simulink library "RF"  (Simulink 4.00)
values from neighbouring files (symbols this model uses):
  A = rms(interp1(f,MX,fb))    [fftbandamp.m]    (also in logfft.m = fftamp(samples, fs, f, varargin{:})/vpp; plotfft.m = fftamp(samples, fs, f, varargin{:})*2/vpp)
  P = sinc((1575.42 - f)/10.23).^2./10.23    [L1PSD.m]    (also in fftphase.m = interp1(f,PX,f0))
undefined symbols (not defined in the file or in its folder): adb, B, CA_ID, fs, j, m, N, p, Phi, Range, Rice_K, Rice_Seed, Rice_Sigma, tau_delay, z
libraries: RF x133, dspcmplx x47, com_sour x8, dspelmat x8, com_chan x4, dspbdsp x3, dspswit x3, simulink_extras x2, com_filt x2
(part 2 of 5)

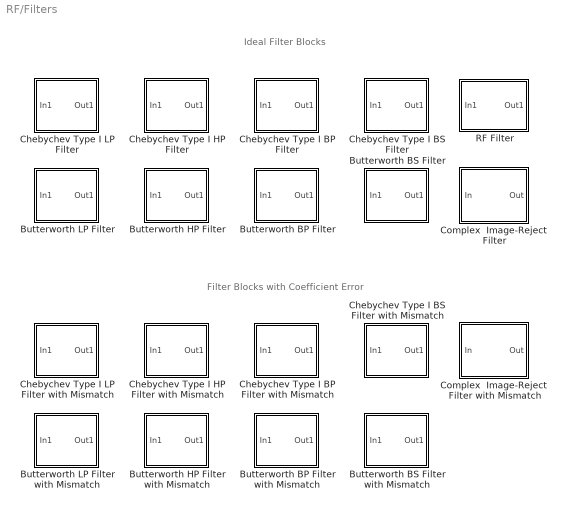
== system RF/Filters ==
  note: Ideal Filter Blocks
  note: Filter Blocks with Coefficient Error
  Butterworth BP Filter : Subsystem  mask(Butterworth Bandpass Filter){w1=200*2*pi, w2=300*2*pi, order=4}
      mask prompts: w1 "Lower Cutoff frequency (rad/sec):"; w2 "Upper Cutoff Frequency"
      mask help: Analog Butterworth bandpass filter.
      mask init:
      | [num,den]=butter(floor(order/2),[w1 w2],'s'); [z,p,k]=tf2zp(num,den); w=logspace(log10(w1/10),log10(10*w2),50);
      | k=k/max(abs(freqs(num,den,w)));[num,den]=zp2tf(z,p,k);h=freqs(num,den,w);
      settings: RTWFcnNameOpts=Auto  RTWFileNameOpts=Auto
      mask Help: Analog Butterworth bandpass filter.
      mask Display: plot(20*log10(w),20*log10(abs(h)))
  Butterworth BP Filter with Mismatch : Subsystem  mask(Butterworth Bandpass Filter with Mismatch){w1=200*2*pi, w2=300*2*pi, order=4, ErrorStd=1}
      mask prompts: w1 "Lower Cutoff frequency (rad/sec):"; w2 "Upper Cutoff Frequency"; ErrorStd "Coefficient Standard Error (Percent Nominal Value)"
      mask help: Analog Butterworth bandpass filter. Coefficient Error is modeled as percent nominal value error.
      mask init:
      | [num,den]=butter(floor(order/2),[w1 w2],'s');[z,p,k]=tf2zp(num,den);
      | w=logspace(log10(w1/10),log10(10*w2),50);
      | k=k/max(abs(freqs(num,den,w))); [num,den]=zp2tf(z,p,k);
      | num = num + num .* ErrorStd/100 .* randn(1,length(num));
      | den = den + den .* ErrorStd/100 .* randn(1,length(den));
      | [z,p,k]=tf2zp(num,den); h=freqs(num,den,w);
      settings: RTWFcnNameOpts=Auto  RTWFileNameOpts=Auto
      mask Help: Analog Butterworth bandpass filter.  Coefficient Error is modeled as percent nominal value error.
      mask Display: plot(20*log10(w),20*log10(abs(h)))
  Butterworth BS Filter : Subsystem  mask(Butterworth Bandstop Filter){w1=100*2*pi, w2=200*2*pi, order=4}
      mask prompts: w1 "Lower Cutoff frequency (rad/sec):"; w2 "Upper Cutoff frequency (rad/sec)"
      mask help: Analog Butterworth bandstop filter.
      mask init:
      | [num,den]=butter(floor(order/2),[w1 w2],'stop','s');[z,p,k]=tf2zp(num,den);
      | w=logspace(log10(w1/10),log10(10*w2),50);
      | k=k/max(abs(freqs(num,den,w)));[num,den]=zp2tf(z,p,k);h=freqs(num,den,w);
      settings: RTWFcnNameOpts=Auto  RTWFileNameOpts=Auto
      mask Help: Analog Butterworth bandstop filter.
      mask Display: plot(20*log10(w),20*log10(abs(h)))
  Butterworth BS Filter with Mismatch : Subsystem  mask(Butterworth Bandstop Filter with Mismatch){w1=100*2*pi, w2=200*2*pi, order=4, ErrorStd=1}
      mask prompts: w1 "Lower Cutoff frequency (rad/sec):"; w2 "Upper Cutoff frequency (rad/sec)"; ErrorStd "Coefficient Standard Error (Percent Nominal Value)"
      mask help: Analog Butterworth bandstop filter. Coefficient Error is modeled as percent nominal value error.
      mask init:
      | [num,den]=butter(floor(order/2),[w1 w2],'stop','s');[z,p,k]=tf2zp(num,den);
      | w=logspace(log10(w1/10),log10(10*w2),50);
      | k=k/max(abs(freqs(num,den,w)));[num,den]=zp2tf(z,p,k);
      | num = num + num .* ErrorStd/100 .* randn(1,length(num));
      | den = den + den .* ErrorStd/100 .* randn(1,length(den));
      | [z,p,k]=tf2zp(num,den); h=freqs(num,den,w);
      settings: RTWFcnNameOpts=Auto  RTWFileNameOpts=Auto
      mask Help: Analog Butterworth bandstop filter.  Coefficient Error is modeled as percent nominal value error.
      mask Display: plot(20*log10(w),20*log10(abs(h)))
  Butterworth HP Filter : Subsystem  mask(Butterworth Highpass Filter){w0=100*2*pi, order=4}
      mask prompts: w0 "Cutoff frequency (rad/sec):"
      mask help: Analog Butterworth highpass filter.
      mask init:
      | [num,den]=butter(order,w0,'high','s');[z,p,k]=tf2zp(num,den);
      | w=logspace(log10(w0/10),log10(10*w0),50);
      | k=k/max(abs(freqs(num,den,w)));[num,den]=zp2tf(z,p,k);h=freqs(num,den,w);
      settings: RTWFcnNameOpts=Auto  RTWFileNameOpts=Auto
      mask Help: Analog Butterworth highpass filter.
      mask Display: plot(20*log10(w),20*log10(abs(h)))
  Butterworth HP Filter with Mismatch : Subsystem  mask(Butterworth Highpass Filter with Mismatch){w0=100*2*pi, order=4, ErrorStd=1}
      mask prompts: w0 "Cutoff frequency (rad/sec):"; ErrorStd "Coefficient Standard Error (Percent Nominal Value)"
      mask help: Analog Butterworth highpass filter. Coefficient Error is modeled as percent nominal value error.
      mask init:
      | [num,den]=butter(order,w0,'high','s');[z,p,k]=tf2zp(num,den);
      | w=logspace(log10(w0/10),log10(10*w0),50);
      | k=k/max(abs(freqs(num,den,w))); [num,den]=zp2tf(z,p,k);
      | num = num + num .* ErrorStd/100 .* randn(1,length(num));
      | den = den + den .* ErrorStd/100 .* randn(1,length(den));
      | [z,p,k]=tf2zp(num,den); h=freqs(num,den,w);
      settings: RTWFcnNameOpts=Auto  RTWFileNameOpts=Auto
      mask Help: Analog Butterworth highpass filter.  Coefficient Error is modeled as percent nominal value error.
      mask Display: plot(20*log10(w),20*log10(abs(h)))
  Butterworth LP Filter : Subsystem  mask(Butterworth Lowpass Filter){w0=100*2*pi, order=4}
      mask prompts: w0 "Cutoff frequency (rad/sec):"
      mask help: Analog Butterworth low pass filter.
      mask init:
      | [num,den]=butter(order,w0,'s');[z,p,k]=tf2zp(num,den);
      | w=logspace(log10(w0/10),log10(10*w0),50);
      | k=k/max(abs(freqs(num,den,w)));[num,den]=zp2tf(z,p,k); h=freqs(num,den,w);
      settings: RTWFcnNameOpts=Auto  RTWFileNameOpts=Auto
      mask Help: Analog Butterworth low pass filter.
      mask Display: plot(20*log10(w),20*log10(abs(h)))
  Butterworth LP Filter with Mismatch : Subsystem  mask(Butterworth Lowpass Filter with Mismatch){w0=100*2*pi, order=4, ErrorStd=1}
      mask prompts: w0 "Cutoff frequency (rad/sec):"; ErrorStd "Coefficient Standard Error (Percent Nominal Value)"
      mask help: Analog Butterworth low pass filter. Coefficient Error is modeled as percent nominal value error.
      mask init:
      | [num,den]=butter(order,w0,'s');[z,p,k]=tf2zp(num,den);
      | w=logspace(log10(w0/10),log10(10*w0),50);
      | k=k/max(abs(freqs(num,den,w)));[num,den]=zp2tf(z,p,k);
      | num = num + num .* ErrorStd/100 .* randn(1,length(num));
      | den = den + den .* ErrorStd/100 .* randn(1,length(den));
      | [z,p,k]=tf2zp(num,den); h=freqs(num,den,w);
      settings: RTWFcnNameOpts=Auto  RTWFileNameOpts=Auto
      mask Help: Analog Butterworth low pass filter.  Coefficient Error is modeled as percent nominal value error.
      mask Display: plot(20*log10(w),20*log10(abs(h)))
  Chebychev Type I BP Filter : Subsystem  mask(Chebychev Type I Bandpass Filter){w1=200*2*pi, w2=300*2*pi, order=4, ripple=0.5}
      mask prompts: w1 "Lower Cutoff frequency (rad/sec):"; w2 "Upper Cutoff frequency (rad/sec)"; ripple "Db ripple in passband:"
      mask help: Analog Chebyshev type I bandpass filter.
      mask init:
      | [z,p,k]=cheby1(floor(order/2),ripple,[w1 w2],'s');
      | [num,den]=zp2tf(z,p,1); w=logspace(log10(w1/10),log10(10*w2),50);
      | k = 1/max(abs(freqs(num,den,w)));[num,den]=zp2tf(z,p,k);
      | h=freqs(num,den,w);
      settings: RTWFcnNameOpts=Auto  RTWFileNameOpts=Auto
      mask Help: Analog Chebyshev type I bandpass filter.
      mask Display: plot(20*log10(w),20*log10(abs(h)))
  Chebychev Type I BP Filter with Mismatch : Subsystem  mask(Chebychev Type I Bandpass Filter with Mismatch){w1=200*2*pi, w2=300*2*pi, order=4, ripple=0.5, ErrorStd=1}
      mask prompts: w1 "Lower Cutoff frequency (rad/sec):"; w2 "Upper Cutoff frequency (rad/sec)"; ripple "Db ripple in passband:"; ErrorStd "Coefficient Standard Error (Percent Nominal Value)"
      mask help: Analog Chebyshev type I bandpass filter. Coefficient Error is modeled as percent nominal value error.
      mask init:
      | [z,p,k]=cheby1(floor(order/2),ripple,[w1 w2],'s');
      | [num,den]=zp2tf(z,p,1); w=logspace(log10(w1/10),log10(10*w2),50);
      | k = 1/max(abs(freqs(num,den,w)));[num,den]=zp2tf(z,p,k);
      | num = num + num .* ErrorStd/100 .* randn(1,length(num));
      | den = den + den .* ErrorStd/100 .* randn(1,length(den));
      | [z,p,k]=tf2zp(num,den); h=freqs(num,den,w);
      settings: RTWFcnNameOpts=Auto  RTWFileNameOpts=Auto
      mask Help: Analog Chebyshev type I bandpass filter.  Coefficient Error is modeled as percent nominal value error.
      mask Display: plot(20*log10(w),20*log10(abs(h)))
  Chebychev Type I BS Filter : Subsystem  mask(Chebychev Type I Bandstop Filter){w1=100*2*pi, w2=200*2*pi, order=4, ripple=0.5}
      mask prompts: w1 "Lower Cutoff frequency (rad/sec):"; w2 "Upper Cutoff frequency (rad/sec)"; ripple "Db ripple in passband:"
      mask help: Analog Chebyshev type I bandstop filter.
      mask init:
      | [z,p,k]=cheby1(floor(order/2),ripple,[w1 w2],'stop','s');
      |  w=logspace(log10(w1/10),log10(10*w2),50);[num,den]=zp2tf(z,p,1);
      | k =1/max(abs(freqs(num,den,w)));[num,den]=zp2tf(z,p,k); h=freqs(num,den,w);
      settings: RTWFcnNameOpts=Auto  RTWFileNameOpts=Auto
      mask Help: Analog Chebyshev type I bandstop filter.
      mask Display: plot(20*log10(w),20*log10(abs(h)))
  Chebychev Type I BS Filter with Mismatch : Subsystem  mask(Chebychev Type I Bandstop Filter with Mismatch){w1=100*2*pi, w2=200*2*pi, order=4, ripple=0.5, ErrorStd=1}
      mask prompts: w1 "Lower Cutoff frequency (rad/sec):"; w2 "Upper Cutoff frequency (rad/sec)"; ripple "Db ripple in passband:"; ErrorStd "Coefficient Standard Error (Percent Nominal Value)"
      mask help: Analog Chebyshev type I bandstop filter. Coefficient Error is modeled as percent nominal value error.
      mask init:
      | [z,p,k]=cheby1(floor(order/2),ripple,[w1 w2],'stop','s');
      |  w=logspace(log10(w1/10),log10(10*w2),50);[num,den]=zp2tf(z,p,1);
      | k =1/max(abs(freqs(num,den,w)));[num,den]=zp2tf(z,p,k);
      | num = num + num .* ErrorStd/100 .* randn(1,length(num));
      | den = den + den .* ErrorStd/100 .* randn(1,length(den));
      | [z,p,k]=tf2zp(num,den);h=freqs(num,den,w);
      settings: RTWFcnNameOpts=Auto  RTWFileNameOpts=Auto
      mask Help: Analog Chebyshev type I bandstop filter.  Coefficient Error is modeled as percent nominal value error.
      mask Display: plot(20*log10(w),20*log10(abs(h)))
  Chebychev Type I HP Filter : Subsystem  mask(Chebychev Type I Highpass Filter){w0=100*2*pi, order=4, ripple=0.5}
      mask prompts: w0 "Cutoff frequency (rad/sec):"; ripple "Db ripple in passband:"
      mask help: Analog Chebyshev type 1 highpass filter.
      mask init:
      | [z,p,k]=cheby1(order,ripple,w0,'high','s');
      | w=logspace(log10(w0/10),log10(10*w0),50);[num,den]=zp2tf(z,p,1);
      | k =1/max(abs(freqs(num,den,w)));[num,den]=zp2tf(z,p,k); h=freqs(num,den,w);
      settings: RTWFcnNameOpts=Auto  RTWFileNameOpts=Auto
      mask Help: Analog Chebyshev type 1 highpass filter.
      mask Display: plot(20*log10(w),20*log10(abs(h)))
  Chebychev Type I HP Filter with Mismatch : Subsystem  mask(Chebychev Type I Highpass Filter with Mismatch){w0=100*2*pi, order=4, ripple=0.5, ErrorStd=1}
      mask prompts: w0 "Cutoff frequency (rad/sec):"; ripple "Db ripple in passband:"; ErrorStd "Coefficient Standard Error (Percent Nominal Value)"
      mask help: Analog Chebyshev type 1 highpass filter. Coefficient Error is modeled as percent nominal value error.
      mask init:
      | [z,p,k]=cheby1(order,ripple,w0,'high','s');
      | w=logspace(log10(w0/10),log10(10*w0),50); [num,den]=zp2tf(z,p,1);
      | k =1/max(abs(freqs(num,den,w))); [num,den]=zp2tf(z,p,k);
      | num = num + num .* ErrorStd/100 .* randn(1,length(num));
      | den = den + den .* ErrorStd/100 .* randn(1,length(den));
      | [z,p,k]=tf2zp(num,den); h=freqs(num,den,w);
      settings: RTWFcnNameOpts=Auto  RTWFileNameOpts=Auto
      mask Help: Analog Chebyshev type 1 highpass filter.  Coefficient Error is modeled as percent nominal value error.
      mask Display: plot(20*log10(w),20*log10(abs(h)))
  Chebychev Type I LP Filter : Subsystem  mask(Chebychev Type I Lowpass Filter){w0=100*2*pi, n=4, ripple=0.5}
      mask prompts: w0 "Cutoff frequency (rad/sec):"; n "Order:"; ripple "Db ripple in passband:"
      mask help: Analog Chebyshev type I low pass filter.
      mask init:
      | [z,p,k]=cheb1ap(n,ripple); z=w0*z; p=w0*p; k=real(prod(-p)); [num,den]=zp2tf(z,p,k); w=logspace(log10(w0/10),log10(10*w0),50); h=freqs(num,den,w);
      settings: RTWFcnNameOpts=Auto  RTWFileNameOpts=Auto
      mask Help: Analog Chebyshev type I low pass filter.
      mask Display: plot(20*log10(w),20*log10(abs(h)))
  Chebychev Type I LP Filter with Mismatch : Subsystem  mask(Chebychev Type I Lowpass Filter with Mismatch){w0=100*2*pi, order=4, ripple=0.5, ErrorStd=1}
      mask prompts: w0 "Cutoff frequency (rad/sec):"; ripple "Db ripple in passband:"; ErrorStd "Coefficient Standard Error (Percent Nominal Value)"
      mask help: Analog Chebyshev type I low pass filter. Coefficient Error is modeled as percent nominal value error.
      mask init:
      | [z,p,k]=cheb1ap(order,ripple); z=w0*z; p=w0*p; k=real(prod(-p));
      | [num,den]=zp2tf(z,p,k);
      | num = num + num .* ErrorStd/100 .* randn(1,length(num));
      | den = den + den .* ErrorStd/100 .* randn(1,length(den));
      | [z,p,k]=tf2zp(num,den);
      | w=logspace(log10(w0/10),log10(10*w0),50); h=freqs(num,den,w);
      settings: RTWFcnNameOpts=Auto  RTWFileNameOpts=Auto
      mask Help: Analog Chebyshev type I low pass filter.  Coefficient Error is modeled as percent nominal value error.
      mask Display: plot(20*log10(w),20*log10(abs(h)))
  Complex  Image-Reject  Filter : Subsystem  mask(Complex Anti-alias Filter){fc=250, f0=100}
      mask prompts: fc "Center Frequency (Hz)"; f0 "Bandwidth (Hz)"
      mask help: 4th Order Continuous Time Complex Bandpass Filter. The filter is a frequency shifted 4th order butterworth lowpass filter.
      mask init:
      | [num,denom] = butter(4,f0*pi,'s');
      | A = num(length(num));
      | p = roots(denom) + j*2*pi*fc;
      | d = real(p);
      | c = imag(p);
      settings: RTWFcnNameOpts=Auto  RTWFileNameOpts=Auto
      mask Help: 4th Order Continuous Time Complex Bandpass Filter.  The filter is a frequency shifted 4th order butterworth lowpass filter.
      mask Display: plot(0,0,100,100,[50,50,90,10],[90,50,50,50],[70,70],[60,50],[80,75,65,60],[50,80,80,49]);
  Complex  Image-Reject  Filter with Mismatch : Subsystem  mask(Complex Anti-alias Filter with Mismatch){fc=250, f0=100, ErrorStd=1}
      mask prompts: fc "Center Frequency (Hz)"; f0 "Bandwidth (Hz)"; ErrorStd "Coefficient Standard Error (Percent Nominal Value)"
      mask help: 4th Order Continuous Time Complex Bandpass Filter. The filter is a frequency shifted 4th order butterworth lowpass filter. Coefficient Error is modeled as percent nominal value error.
      mask init:
      | [num,denom] = butter(4,f0*pi,'s');
      | A = num(length(num));
      | p = roots(denom) + j*2*pi*fc;
      | d = real(p);
      | c = imag(p);
      | 
      | d1 = d + d .* ErrorStd/100 .* randn(length(d),1);
      | d2 = d + d .* ErrorStd/100 .* randn(length(d),1);
      | c1 = c + c .* ErrorStd/100 .* randn(length(c),1);
      | c2 = c + c .* ErrorStd/100 .* randn(length(c),1);
      settings: RTWFcnNameOpts=Auto  RTWFileNameOpts=Auto
      mask Help: 4th Order Continuous Time Complex Bandpass Filter.  The filter is a frequency shifted 4th order butterworth lowpass filter.  Coefficient Error is modeled as percent nominal value error.
      mask Display: plot(0,0,100,100,[50,50,90,10],[90,50,50,50],[70,70],[60,50],[80,75,65,60],[50,80,80,49]);
  RF Filter : Subsystem  mask(RF Passive Bandpass Filter){Q=5, f0=1575.42E6, n=1, Gi=1}
      mask prompts: f0 "Band Center (Hz)"; n "Number of stages"; Gi "Interstage Gain (absolute)"
      mask help: RF Passive Bandpass Filter. All stages have band center at the signal center frequency.
      mask init:
      | w0 = 2*pi*f0;denom = [1 w0/Q w0^2];
      | for temp = 1:n-1,
      |   denom = conv(denom,[1 w0/Q w0^2]);
      |  end;
      | num = [(Gi*w0*Q)^n zeros(1,n)];
      | w=logspace(log10(w0/10),log10(10*w0),50); h=freqs(num,denom,w);
      settings: RTWFcnNameOpts=Auto  RTWFileNameOpts=Auto
      mask Help: RF Passive Bandpass Filter.  All stages have band center at the signal center frequency.
      mask Display: plot(20*log10(w),20*log10(abs(h)))

== system RF/GPS Blocks ==
  note: Global Positioning System (GPS) Specific Blocks
  note: Global Positioning System (GPS) Receiver Blocks
  "C/A Code, 1.023MHz" : Subsystem  mask(CA Sequence){CA_PRN_ID=CA_ID}
      mask prompts: CA_PRN_ID "CA ID"
      mask help: CA pseudo-noise sequence for CDMA transmission of GPS navigation data. CA ID is an integer in the range 1 - 32 which selects a unique phase of the code. Data rate is 1.023 MHz.
      mask init:
      | [x,y]=srcsicon(5);
      settings: RTWFcnNameOpts=Auto  RTWFileNameOpts=Auto
      mask Help: CA pseudo-noise sequence for CDMA transmission of GPS navigation data.  CA ID is an integer in the range 1 - 32 which selects a unique phase of the code.  Data rate is 1.023 MHz.
      mask Display: plot(0,0,100,100,x,y);disp('CA Sequence ')
  Co-channel Interference : Subsystem  mask(GPS Co-channel Interference){d=[], CA=[1 2 3 4 5 6], Seeds=[1 2 3 4 5 6 ], Rice_Seeds=[7 8 9 10 11 12], AWGN_Seeds=[13 14 15 16 17 18], P_Seeds=[19 20 21 22 23 24], taus_delay=[], taus=[]}
      mask prompts: d "Distances (from SV)"; CA "Satellite CA Codes"; Seeds "Navigation Data Seeds"; Rice_Seeds "Rice Seeds"; AWGN_Seeds "AWGN Seeds"; P_Seeds "P Code Seeds"; taus_delay "Delay Spreads"; taus "Atmospheric Delays"
      mask help:
      | GPS Co-channel interference.  Interference by satellite transmitters other than the transmitter to be received.
      |
      | This block is unfinished, and essentially untested.
      settings: RTWFcnNameOpts=Auto  RTWFileNameOpts=Auto
      mask Help:
      | GPS Co-channel interference.  Interference by satellite transmitters other than the transmitter to be received.
      | 
      | This block is unfinished, and essentially untested.
      mask Display:
      | plot(0,0,100,100,[95 5 10 10 10 (100-15)*[0:1/30:1]+10],[75 75 75 70 95 rand(1,31)*20+75]);
      | disp('Co-Channel Interference')
  Direct Conversion Receiver : Subsystem  mask(GPS Receiver: Direct Conversion){FPError=, SDPError=}
      mask prompts: FPError "Filter Mismatch (Percent Nominal Value)"; SDPError "Sigma-Delta Mismatch (Percent Nominal Value)"
      mask help:
      | GPS Receiver using a Direct Conversion architecture.  The receiver models nonidealities in the LNA, mixer, and A/D converter, as well as amplitude and phase distortion between the quadrature paths.  The output is a complex signal of the form I(t)+j*Q(t).
      |
      | This block is unfinished, and essentially untested.
      settings: RTWFcnNameOpts=Auto  RTWFileNameOpts=Auto
      mask Help:
      | GPS Receiver using a Direct Conversion architecture.  The receiver models nonidealities in the LNA, mixer, and A/D converter, as well as amplitude and phase distortion between the quadrature paths.  The output is a complex signal of the form I(t)+j*Q(t).
      | 
      | This block is unfinished, and essentially untested.
      mask Display:
      | plot(0,0,100,100,[5+1.5*[[0:.8:10] [10:0.8:20] [20:.8:30]] 50 50 50 50+15*[0 1 1 2 2 3]],[85+10*[sin([0:.8:10]*pi*2/5) sin([10:0.8:20]*pi*2/5-pi) sin([20:.8:30]*pi*2/5)] 85 99 75 85+8*[1 1 -1 -1 1 1]]);
      | disp('GPS Receiver')
  GPS Channel : Subsystem  mask(GPS RF Channel){Rice_Seed=1, tau_delay=, AWGN_Seed=12345, d=, tau=}
      mask prompts: Rice_Seed "Rician Fading Seed"; tau_delay "Delay Spread"; AWGN_Seed "White Noise Seed"; d "Distance from SV"; tau "Atmospheric Delay"
      mask help:
      | RF transmission channel with white noise, impulse noise, and
      | large-scale and small scale fading.
      |
      | This block is unfinished, and essentially untested.
      mask init:
      | d_ref = ;
      | v_ref = ;
      | sigma_signal = ;
      | n = 4;
      | Rice_Sigma = ;
      | Rice_K = ;
      | AWGN_Mean = 0;
      | AWGN_Variance = ;
      | Pulse_Prob =;
      | Pulse_Duration =;
      | Pulse_Sigma =;
      | Pulse_Amp =;
      | Pulse_Poles =;
      | Pulse_Zeros =;
      settings: RTWFcnNameOpts=Auto  RTWFileNameOpts=Auto
      mask Help:
      | RF transmission channel with white noise, impulse noise, and
      | large-scale and small scale fading.
      | 
      | This block is unfinished, and essentially untested.
      mask Display:
      | plot(0,0,100,100,[05 15 10 10 05 10 18 14 13 7.5 13 41 44 47 50 53 57 59 100-[13 7.5 13 14 18 10 5 10 10 15 5]],[70 70 70 85 92 85 79 82 90 88.5 90 90 87 93 87 93 87 90 90 88.5 90 82 79 85 92 85 70 70 70]);
      | disp('GPS Channel')
  GPS Transmitter : Subsystem  mask(GPS SV Transmitter){tsrf=1/48/1575.42E6, CA_ID=3, P_Seed=157}
      mask prompts: tsrf "RF Sample Time"; CA_ID "Satellite CA ID"; P_Seed "P Code Seed"
      mask help:
      | GPS SV Transmitter Block.  Input port for navigation data (at 50 Hz).  Satellite ID(1 - 32) and sample rate are variable.  Data is modulated by a CA code based on the satellite ID (at 1.023 MHz) and by a randomly generated P code (at 10.23 MHz).  This resulting sequence is BPSK modulated to form the L1 output.  The carrier is at 1575.42 MHz.
      |
      | This block is unfinished, and essentially untested.
      settings: RTWFcnNameOpts=Auto  RTWFileNameOpts=Auto
      mask Help:
      | GPS SV Transmitter Block.  Input port for navigation data (at 50 Hz).  Satellite ID(1 - 32) and sample rate are variable.  Data is modulated by a CA code based on the satellite ID (at 1.023 MHz) and by a randomly generated P code (at 10.23 MHz).  This resulting sequence is BPSK modulated to form the L1 output.  The carrier is at 1575.42 MHz.
      | 
      | This block is unfinished, and essentially untested.
      mask Display:
      | plot(0,0,100,100,[5+15*[0 1 1 2 2 3] 50 50 50 50+1.5*[[0:.8:10] [10:.8:20] [20:.8:30]]],[85+8*[1 1 -1 -1 1 1] 85 99 75 85+10*[sin([0:.8:10]*pi*2/5) sin([10:.8:20]*pi*2/5 - pi) sin([20:.8:30]*pi*2/5)]]);
      | disp('GPS SV TX')
  Low IF Receiver : Subsystem  mask(GPS Receiver: Low IF){FPError=, SDPError=}
      mask prompts: FPError "Filter Mismatch (Percent Nominal Value)"; SDPError "Sigma-Delta Mismatch (Percent Nominal Value)"
      mask help:
      | GPS Receiver using a Low IF architecture.  The receiver models nonidealities in the LNA, mixer, and A/D converter, as well as amplitude and phase distortion between the quadrature paths.  The output is a complex signal of the form I(t)+j*Q(t).
      |
      | This block is unfinished, and essentially untested.
      settings: RTWFcnNameOpts=Auto  RTWFileNameOpts=Auto
      mask Help:
      | GPS Receiver using a Low IF architecture.  The receiver models nonidealities in the LNA, mixer, and A/D converter, as well as amplitude and phase distortion between the quadrature paths.  The output is a complex signal of the form I(t)+j*Q(t).
      | 
      | This block is unfinished, and essentially untested.
      mask Display:
      | plot(0,0,100,100,[5+1.5*[[0:.8:10] [10:0.8:20] [20:.8:30]] 50 50 50 50+15*[0 1 1 2 2 3]],[85+10*[sin([0:.8:10]*pi*2/5) sin([10:0.8:20]*pi*2/5-pi) sin([20:.8:30]*pi*2/5)] 85 99 75 85+8*[1 1 -1 -1 1 1]]);
      | disp('GPS Receiver')
  Low IF Receiver with  QBP Sigma-Delta : Subsystem  mask(GPS Receiver: Low IF with QBPSD){FPError=, SDPError=}
      mask prompts: FPError "Filter Mismatch (Percent Nominal Value)"; SDPError "Sigma-Delta Mismatch (Percent Nominal Value)"
      mask help:
      | GPS Receiver using a Low IF with Quadrature Bandpass Sigma-Delta Modulator architecture as described by Stephen Jantzi, "Quadrature Bandpass Delta-Sigma Modulation for Digital Radio," Ph.D. dissertation, University of Toronto.  The receiver models nonidealities in the LNA, mixer, and A/D converter, as well as amplitude and phase distortion between the quadrature paths.  The output is a complex signal of the form I(t)+j*Q(t).
      |
      | This block is unfinished, and essentially untested.
      settings: RTWFcnNameOpts=Auto  RTWFileNameOpts=Auto
      mask Help:
      | GPS Receiver using a Low IF with Quadrature Bandpass Sigma-Delta Modulator architecture as described by Stephen Jantzi, "Quadrature Bandpass Delta-Sigma Modulation for Digital Radio," Ph.D. dissertation, University of Toronto.  The receiver models nonidealities in the LNA, mixer, and A/D converter, as well as amplitude and phase distortion between the quadrature paths.  The output is a complex signal of the form I(t)+j*Q(t).
      | 
      | This block is unfinished, and essentially untested.
      mask Display:
      | plot(0,0,100,100,[5+1.5*[[0:.8:10] [10:0.8:20] [20:.8:30]] 50 50 50 50+15*[0 1 1 2 2 3]],[85+10*[sin([0:.8:10]*pi*2/5) sin([10:0.8:20]*pi*2/5-pi) sin([20:.8:30]*pi*2/5)] 85 99 75 85+8*[1 1 -1 -1 1 1]]);
      | disp('GPS Receiver')
  Navigation Data : Subsystem  mask(Random Navigation Data){Seed=1}
      mask prompts: Seed "Random Seed"
      mask help: Random binary data output at 50Hz to approximate GPS navigation data.
      mask init:
      | [x,y]=srcsicon(5);
      settings: RTWFcnNameOpts=Auto  RTWFileNameOpts=Auto
      mask Help: Random binary data output at 50Hz to approximate GPS navigation data.
      mask Display: plot(0,0,100,100,x,y);disp('Navigation Data')

== system RF/Miscellaneous ==
  note: Miscellaneous Useful Blocks
  Clocked  Integrator : Subsystem  TreatAsAtomicUnit=on
      settings: RTWFcnNameOpts=Auto  RTWFileNameOpts=Auto
      mask Type: Clocked Integrator
      mask Description: Clocked Integrator
      mask Help: Clocked Integrator
      mask Display: plot(0,0,100,100,[60,70,20,40,20,70,60],[70,90,90,50,10,10,30])
  Clocked Delaying Integrator : Subsystem  TreatAsAtomicUnit=on
      settings: RTWFcnNameOpts=Auto  RTWFileNameOpts=Auto
      mask Type: Clocked Delaying Integrator
      mask Description: Clocked Delaying Integrator
      mask Help: Clocked Delaying Integrator
      mask Display: plot(0,0,100,100,[60,70,20,40,20,70,60],[70,90,90,50,10,10,30])
  Inverse dB : Subsystem  mask(Inverse dB){intype=Amplitude}
      mask prompts: intype "Input signal:"
      mask help: Convert input from dB.
      mask init:
      | g=10*intype;
      settings: RTWFcnNameOpts=Auto  RTWFileNameOpts=Auto
      mask Help: Convert input from dB.
      mask StyleString: popup(Power|Amplitude)
      mask Display: disp('AdB')
  Linear : Subsystem  mask(Linear Function){Gain=Range/(2^m-1), Offset=-Range/2}
      mask help: Implements Y = Gain*X + Offset
      settings: RTWFcnNameOpts=Auto  RTWFileNameOpts=Auto
      mask Help: Implements Y = Gain*X + Offset
      mask Display: plot(0,0,100,100,[50,50],[10,90],[90,10],[50,50],[90,80,60,40,20],[45,40,30,20,10])
  Maximum Magnitude Switch : Subsystem
      settings: RTWFcnNameOpts=Auto  RTWFileNameOpts=Auto
      mask Type: Maximum Magnitude Switch
      mask Description: Selects the input with the maximum magnitude.
      mask Help: Selects the input with the maximum magnitude.
      mask Display: disp('Max |*|')
  Minimum Magnitude Switch : Subsystem
      settings: RTWFcnNameOpts=Auto  RTWFileNameOpts=Auto
      mask Type: Minimum Magnitude Switch
      mask Description: Selects the input with the minimum magnitude.
      mask Help: Selects the input with the minimum magnitude.
      mask Display: disp('Min |*|')
  N-Sample Switch w/Reset : Subsystem  TreatAsAtomicUnit=on  mask(N-Sample Switch with Reset){N=8, Ts=1}
      mask prompts: N "Switch count, N:"; Ts "Sample time:"
      mask help: Output N samples from the top port. Thereafter, output samples from the bottom port. Resettable.
      mask init:
      | S=12; t=(0:S)/S*2*pi; a=0.05; xc=a*cos(t); yc=a*sin(t);
      | xc4=[xc+.45 NaN xc+.45 NaN xc+.8];
      | yc4=[yc+3/4 NaN yc+1/4 NaN yc+.5];
      | x=[ .85 1 NaN 0 .4       NaN   0 .4      NaN .75 .525 NaN .595 .525 .55];
      | y=[ .5 .5 NaN 3/4 3/4 NaN 1/4 1/4 NaN .5 .7       NaN .7 .7 .61];
      | xs=[xc(4:9) xc(9)+[-.03 0 -.01] ]*3.5+.8;
      | ys=[yc(4:9) yc(9)+[0.01 0 .03 ] ]*3.5+.5;
      settings: RTWFcnNameOpts=Auto  RTWFileNameOpts=Auto
      mask Help: Output N samples from the top port.  Thereafter, output samples from the bottom port. Resettable.
      mask Display:
      | plot(xc4,yc4, xs,ys, x,y);
      | text(1, 0.05, num2str(N),'horiz','right','vert','base');
  PFD : Subsystem
      settings: RTWFcnNameOpts=Auto  RTWFileNameOpts=Auto
      mask Type: Phase/Frequency Detector
      mask Description: Phase/Frequency Detector as described in RF Microelectronics by Behzad Razavi on page 260.
      mask Help: Phase/Frequency Detector as described in RF Microelectronics by Behzad Razavi on page 260.

== system RF/Model Nonidealities ==
  note: Blocks for Modeling Circuit Nonidealities
  Amplitude and Phase Error : Subsystem  mask(Amplitude and Phase Error){A=1.001, tau=100*1/360}
      mask prompts: A "Gain"; tau "Delay"
      mask help: Multiplies the amplitude by a fixed constant, and delays the signal by a fixed time. Used to model amplitude and phase mismatch between quadrature signal paths. Due to innacuracy in the built-in delay block, the delay should be at least as long as the simulation step size.
      settings: RTWFcnNameOpts=Auto  RTWFileNameOpts=Auto
      mask Help: Multiplies the amplitude by a fixed constant, and delays the signal by a fixed time.  Used to model amplitude and phase mismatch between quadrature signal paths.  Due to innacuracy in the built-in delay block, the delay should be at least as long as the simulation step size.
      mask Display: plot([-1:1/8:1]*0.75,sin(0:pi/8:2*pi),[-0.5:1/8:1.5]*0.75,sin(0:pi/8:2*pi)*0.75)
  Compression : Subsystem  mask(Compression){V1dB=-4}
      mask prompts: V1dB "1 dB Compression Amplitude (dbV)"
      mask help: Implements large-signal compresssion. The 1 dB compression point is the input amplitude at which the output amplitude is compressed by 1 dB. A simple tanh function has a 1 dB compression point of -4 dB.
      mask init:
      | Adjust = V1dB + 4;
      settings: RTWFcnNameOpts=Auto  RTWFileNameOpts=Auto
      mask Help: Implements large-signal compresssion.  The 1 dB compression point is the input amplitude at which the output amplitude is compressed by 1 dB.  A simple tanh function has a 1 dB compression point of -4 dB.
      mask Display: plot(0,0,100,100,[50,50],[100,0],[100,0],[50,50],[100,90,80,70,50,30,20,10,0],[100,100,99,95,49,4,1,0,0])
  Flicker Noise : Subsystem  mask(Flicker Noise){f0=1000, N0=1.147E-7, fm=10E3, numtaps=100, Seed=3}
      mask prompts: f0 "Reference Frequency (Hz)"; N0 "Reference Noise Amplitude (V/Hz^0.5)"; fm "Maximum Frequency of Interest"; numtaps "Number of Taps"; Seed "Noise Seed"
      mask help: Flicker Noise: Generates Noise with a PSD inversely proportional to frequency. The noise generation algorithm is to pass white noise through a FIR filter whose frequency response is proportional to 1/sqrt(f). The algorithm is due to N. J. Kasdin, "Discrete Simulation of Colored Noise and Stochastic Processes and 1/f^a Power Law Noise Generation," Proceedings of the IEEE, May 1995, and the implementation is based on that by Jeff Schenk. The valid frequency range is from 1/(N*ts), where N is the number of taps and ts is the sampling time, to fs/2. Below the former, the PSD is constant.
      mask init:
      | a=zeros(1,numtaps); a(1)=1;
      | for temp=2:numtaps,
      |   a(temp)=(temp-2.5)*a(temp-1)/(temp-1);
      | end;
      | ts=1/2/fm;
      | g=sqrt(2*pi*f0*N0^2);
      settings: RTWFcnNameOpts=Auto  RTWFileNameOpts=Auto
      mask Help: Flicker Noise: Generates Noise with a PSD inversely proportional to frequency.  The noise generation algorithm is to pass white noise through a FIR filter whose frequency response is proportional to 1/sqrt(f).  The algorithm is due to N. J. Kasdin, "Discrete Simulation of Colored Noise and Stochastic Processes and 1/f^a Power Law Noise Generation," Proceedings of the IEEE, May 1995, and the implementation is based on that by Jeff Schenk.  The valid frequency range is from 1/(N*ts), where N is the number of taps and ts is the sampling time, to fs/2.  Below the former, the PSD is constant.
      mask Display: plot(0,0,100,100,[10,10],[0,100],[100,0],[10,10],[100,90,10],[20,20,90])
  Nonlinear TF : Subsystem  mask(Nonlinear Transfer Function){Gain1=0, IIP2=40, IIP3=10}
      mask prompts: Gain1 "Primary Gain (dB)"; IIP2 "Second Order Intercept (dB)"; IIP3 "Third Order Intercept(dB)"
      mask help: Implements small signal non-linearity. Only the fundamental, quadratic, and cubic terms are modeled. The intercept points are the input amplitudes at which the intermodulation product coefficients are the same size as the fundamental coefficients.
      mask init:
      | Gain2 = -(Gain1 + IIP2);
      | Gain3 = -2 * (Gain1 + IIP3);
      settings: RTWFcnNameOpts=Auto  RTWFileNameOpts=Auto
      mask Help: Implements small signal non-linearity.  Only the fundamental, quadratic, and cubic terms are modeled.  The intercept points are the input amplitudes at which the intermodulation product coefficients are the same size as the fundamental coefficients.
      mask Display: plot(0,0,100,100,[10,10],[90,10],[90,0],[20,20],[20,20],[70,20],[40,40],[40,20],[80,80],[30,20])

== system RF/Transmission  Channel Blocks ==
  note: Blocks for Modeling Transmission Channel
  Doppler Fading Envelope : Subsystem  mask(Doppler Fading){fm=20, N=1024, NVar=1}
      mask prompts: fm "Maximum Doppler Frequency"; N "Number FFT points"; NVar "White Noise Variance"
      mask help: Doppler Fading Envelope as described in Wireless Communication, Principles and Practice, Theodore Rappaport, Prentice Hall. Implemented using FFT and IFFT.
      mask init:
      | ts=1/2/fm;del_f=2*fm/(N-1);f=[-fm+del_f:del_f:fm-del_f];
      | H = sqrt(1.5/pi/fm./sqrt(1-(f/fm).^2));
      | H = fftshift([2*H(1)-H(2) H 2*H(length(H))-H(length(H)-1)]);
      | t = rot90((0:2*N-1)/del_f/N,-1);
      | IC1=[real(ifft(fft(NVar*randn(1,N)).*H)) real(ifft(fft(NVar*randn(1,N)).*H))];
      | IC2=[real(ifft(fft(NVar*randn(1,N)).*H)) real(ifft(fft(NVar*randn(1,N)).*H))];
      | IC1=[t rot90(IC1,-1)]; IC2=[t rot90(IC2,-1)];
      settings: RTWFcnNameOpts=Auto  RTWFileNameOpts=Auto
      mask Help: Doppler Fading Envelope as described in Wireless Communication, Principles and Practice, Theodore Rappaport, Prentice Hall.  Implemented using FFT and IFFT.
      mask Display: plot([-fm:2*fm/(N-1):fm],fftshift(H))
  Doppler Fading with User Defined Filter : Subsystem  mask(Doppler Fading){NVar=1, Seed=[1 5 7 2], Num=[1], Denom=[1], ts=1/1E6}
      mask prompts: NVar "White Noise Variance"; Seed "Noise Seeds (4 integers)"; Num "Filter Numerator"; Denom "Filter Denominator"; ts "Filter Sample Time"
      mask help: Doppler Fading using a user supplied baseband complex doppler filter.
      settings: RTWFcnNameOpts=Auto  RTWFileNameOpts=Auto
      mask Help: Doppler Fading using a user supplied baseband complex doppler filter.
      mask Display: disp('Doppler Fading')
  Doppler and  Multi-path Fading : Subsystem  mask(Multipath Fading Assuming a LOS Path){seed=Rice_Seed, sigma=Rice_Sigma, K=Rice_K, DelaySpread=tau_delay}
      mask prompts: K "Rician K-factor"; DelaySpread "Delay Spread"
      mask help: Multipath Fading assuming a LOS transmission path as well as Doppler fading as described in Wireless Communications, Principles and Practice, Theodore Rappaport, Prentice Hall.
      settings: RTWFcnNameOpts=Auto  RTWFileNameOpts=Auto
      mask Help: Multipath Fading assuming a LOS transmission path as well as Doppler fading as described in Wireless Communications, Principles and Practice, Theodore Rappaport, Prentice Hall.
      mask Display:
      | plot(0,0,100,100,[95 5 10 10 10 (100-15)*[0:1/30:1]+10],[75 75 75 70 95 rand(1,31)*20+75]);
      | disp('Rician Fading')
  Exponential Path Loss and Log-Normal Shadowing : Subsystem  mask(Log-Normal Shadowing and Exponential Path Loss){d0=1, d=1E4, p0=1, Sigma_P=1, n=3}
      mask prompts: d0 "Reference Distance"; d "Transmitter Distance"; p0 "Reference Signal Level"; Sigma_P "Signal Level Variance"; n "Path Loss Exponent"
      mask help: Log-Normal Shadowing and Exponential Path Loss as described in Wireless Communications, Principles & Practice, Theodore Rappaport, Prentice Hall.
      settings: RTWFcnNameOpts=Auto  RTWFileNameOpts=Auto
      mask Help: Log-Normal Shadowing and Exponential Path Loss as described in Wireless Communications, Principles & Practice, Theodore Rappaport, Prentice Hall.
      mask Display:
      | plot(0,0,100,100,[95 5 10 10 10 (100-15)*[0:1/30:1]+10],[75 75 75 70 95 rand(1,31)*20+75]);
      | disp('Log-Normal')
  Impulse Noise : Subsystem  mask(Impulse Noise Generator){P_Impulse=1/1000, T_Impulse=1/1E6, Amp_Var=1, Amp_Mean=0.25, Num=[], Denom=[]}
      mask prompts: P_Impulse "Likelihood"; T_Impulse "Sample Time"; Amp_Var "Amplitude Variance"; Amp_Mean "Mean Amplitude"; Num "Filter Numerator"; Denom "Filter Denominator"
      mask help: Generates impulse noise of mean amplitude, duration, and likelihood given by the block parameters. Impulse is filtered by specified filter to give the desired pulse shape.
      settings: RTWFcnNameOpts=Auto  RTWFileNameOpts=Auto
      mask Help: Generates impulse noise of mean amplitude, duration, and likelihood given by the block parameters.  Impulse is filtered by specified filter to give the desired pulse shape.
      mask Display:
      | plot(0,0,100,100,[80,80,90,10],[90,80,80,80],[10,10],[85,80],[14,14],[74,80],[50,50],[95,80]);
      | disp('Impulse Noise');
  Out-of-Band  Interference : Subsystem  mask(Interference){fo=200, fbw=20, Ripple=0.5, Order=8, Frequencies=[0], Amplitudes=[0], Phases=[0], AWGNVRMS=0.25, AWGNSeed=4}
      mask prompts: fo "Band Center (Hz)"; fbw "Band Width (Hz)"; Ripple "Ripple (dB)"; Order "Filter Order"; Frequencies "Tone Frequencies (rads/sec)"; Amplitudes "Tone Amplitudes"; Phases "Tone Phases (radians)"; AWGNVRMS "Noise RMS Voltage"; AWGNSeed "Noise Seed"
      mask help: Generates out-of-band noise and tones. The noise is bandstop filtered to prevent in-band noise. Any number of tones can be added by using a matrix for the tone parameters.
      settings: RTWFcnNameOpts=Auto  RTWFileNameOpts=Auto
      mask Help: Generates out-of-band noise and tones.  The noise is bandstop filtered to prevent in-band noise.  Any number of tones can be added by using a matrix for the tone parameters.
      mask Display:
      | plot(0,0,100,100,[95 5 10 10 10 (100-15)*[0:1/30:1]+10],[75 75 75 70 95 rand(1,31)*20+75]);
      | disp('Interference')

== system RF/A/D Blocks/2nd Order Decimation Filter1 ==
  Data In : Inport  Port=1
  Downsample : dspbdsp/Downsample  N=N  phase=0  ts=1/fs
  Second-Order Integrator : RF/A//D Blocks/Second-Order Integrator  fs=fs  N=N
  Data Out : Outport  Port=1  InitialOutput=0
  wires:
  Downsample/1 -> Data Out/1
  Second-Order Integrator/1 -> Downsample/1
  Data In/1 -> Second-Order Integrator/1

== system RF/A/D Blocks/3rd Order Decimation Filter ==
  Data In : Inport  Port=1
  Downsample : dspbdsp/Downsample  N=N  phase=0  ts=1/fs
  Third-Order Integrator : RF/A//D Blocks/Third-Order Integrator  fs=fs  N=N
  Data Out : Outport  Port=1  InitialOutput=0
  wires:
  Downsample/1 -> Data Out/1
  Third-Order Integrator/1 -> Downsample/1
  Data In/1 -> Third-Order Integrator/1

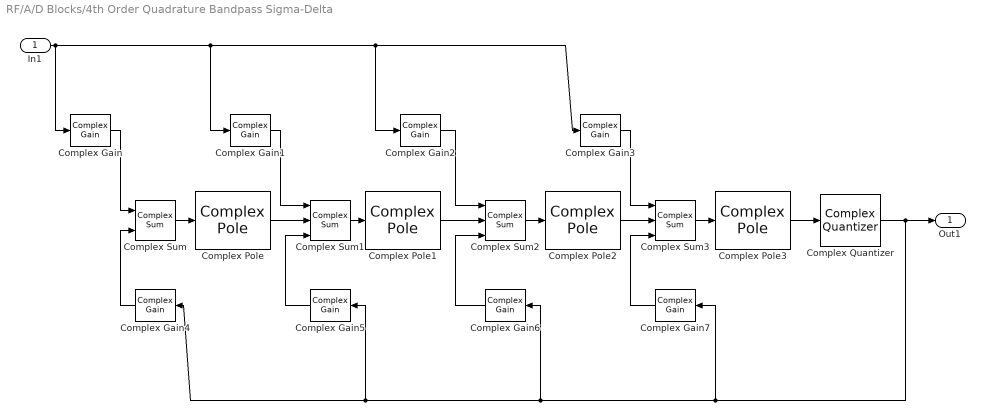
== system RF/A/D Blocks/4th Order Quadrature Bandpass Sigma-Delta ==
  In1 : Inport  Port=1
  Complex Gain : RF/Complex Blocks/Complex Gain  G=A(1)
  Complex Gain1 : RF/Complex Blocks/Complex Gain  G=A(2)
  Complex Gain2 : RF/Complex Blocks/Complex Gain  G=A(3)
  Complex Gain3 : RF/Complex Blocks/Complex Gain  G=A(4)
  Complex Gain4 : RF/Complex Blocks/Complex Gain  Orientation=left  G=B(1)
  Complex Gain5 : RF/Complex Blocks/Complex Gain  Orientation=left  G=B(2)
  Complex Gain6 : RF/Complex Blocks/Complex Gain  Orientation=left  G=B(3)
  Complex Gain7 : RF/Complex Blocks/Complex Gain  Orientation=left  G=B(4)
  Complex Quantizer : RF/Complex Blocks/Complex Quantizer  L_Out_C=-1  H_Out_C=1  Bound_C=0
  Complex Pole : RF/Complex Blocks/Complex Pole  c=c(1)  d=d(1)  ts=ts
  Complex Pole1 : RF/Complex Blocks/Complex Pole  c=c(2)  d=d(2)  ts=ts
  Complex Pole2 : RF/Complex Blocks/Complex Pole  c=c(3)  d=d(3)  ts=ts
  Complex Pole3 : RF/Complex Blocks/Complex Pole  c=c(4)  d=d(4)  ts=ts
  Complex Sum : dspcmplx/Complex Sum  Inputs=++
  Complex Sum1 : dspcmplx/Complex Sum  Inputs=+++
  Complex Sum2 : dspcmplx/Complex Sum  Inputs=+++
  Complex Sum3 : dspcmplx/Complex Sum  Inputs=+++
  Out1 : Outport  Port=1  InitialOutput=0
  wires:
  Complex Quantizer/1 -> Complex Gain4/1, Complex Gain5/1, Complex Gain6/1, Complex Gain7/1, Out1/1
  Complex Pole3/1 -> Complex Quantizer/1
  Complex Sum3/1 -> Complex Pole3/1
  Complex Gain2/1 -> Complex Sum2/1
  Complex Gain3/1 -> Complex Sum3/1
  Complex Sum2/1 -> Complex Pole2/1
  Complex Gain6/1 -> Complex Sum2/3
  Complex Gain7/1 -> Complex Sum3/3
  Complex Pole1/1 -> Complex Sum2/2
  Complex Pole2/1 -> Complex Sum3/2
  Complex Sum/1 -> Complex Pole/1
  Complex Gain5/1 -> Complex Sum1/3
  In1/1 -> Complex Gain2/1, Complex Gain3/1, Complex Gain1/1, Complex Gain/1
  Complex Gain1/1 -> Complex Sum1/1
  Complex Gain/1 -> Complex Sum/1
  Complex Sum1/1 -> Complex Pole1/1
  Complex Pole/1 -> Complex Sum1/2
  Complex Gain4/1 -> Complex Sum/2

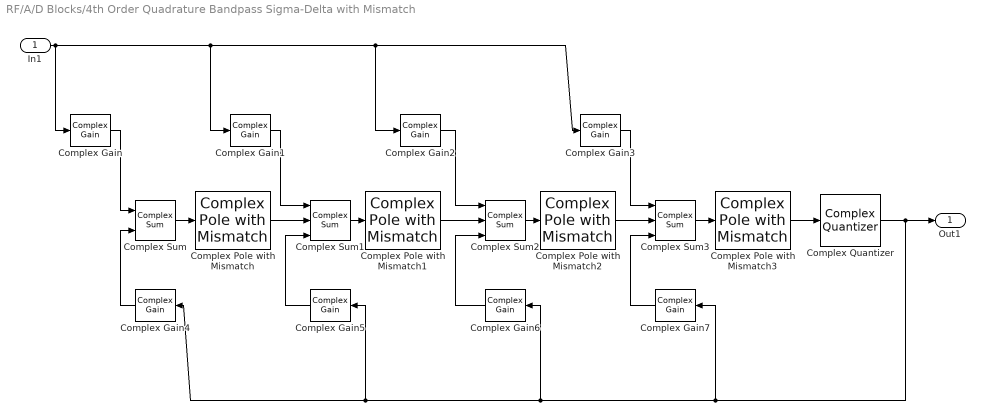
== system RF/A/D Blocks/4th Order Quadrature Bandpass Sigma-Delta with Mismatch ==
  In1 : Inport  Port=1
  Complex Gain : RF/Complex Blocks/Complex Gain  G=A(1)
  Complex Gain1 : RF/Complex Blocks/Complex Gain  G=A(2)
  Complex Gain2 : RF/Complex Blocks/Complex Gain  G=A(3)
  Complex Gain3 : RF/Complex Blocks/Complex Gain  G=A(4)
  Complex Gain4 : RF/Complex Blocks/Complex Gain  Orientation=left  G=B(1)
  Complex Gain5 : RF/Complex Blocks/Complex Gain  Orientation=left  G=B(2)
  Complex Gain6 : RF/Complex Blocks/Complex Gain  Orientation=left  G=B(3)
  Complex Gain7 : RF/Complex Blocks/Complex Gain  Orientation=left  G=B(4)
  Complex Quantizer : RF/Complex Blocks/Complex Quantizer  L_Out_C=-1  H_Out_C=1  Bound_C=0
  Complex Pole with Mismatch : RF/Complex Blocks/Complex Pole with Mismatch  c1=c1(1)  c2=c2(1)  d1=d1(1)  d2=d2(1)  ts=ts
  Complex Pole with Mismatch1 : RF/Complex Blocks/Complex Pole with Mismatch  c1=c1(2)  c2=c2(2)  d1=d1(2)  d2=d2(2)  ts=ts
  Complex Pole with Mismatch2 : RF/Complex Blocks/Complex Pole with Mismatch  c1=c1(3)  c2=c2(3)  d1=d1(3)  d2=d2(3)  ts=ts
  Complex Pole with Mismatch3 : RF/Complex Blocks/Complex Pole with Mismatch  c1=c1(4)  c2=c2(4)  d1=d1(4)  d2=d2(4)  ts=ts
  Complex Sum : dspcmplx/Complex Sum  Inputs=++
  Complex Sum1 : dspcmplx/Complex Sum  Inputs=+++
  Complex Sum2 : dspcmplx/Complex Sum  Inputs=+++
  Complex Sum3 : dspcmplx/Complex Sum  Inputs=+++
  Out1 : Outport  Port=1  InitialOutput=0
  wires:
  Complex Gain4/1 -> Complex Sum/2
  Complex Pole with Mismatch/1 -> Complex Sum1/2
  Complex Sum1/1 -> Complex Pole with Mismatch1/1
  Complex Gain/1 -> Complex Sum/1
  Complex Gain1/1 -> Complex Sum1/1
  In1/1 -> Complex Gain/1, Complex Gain1/1, Complex Gain3/1, Complex Gain2/1
  Complex Gain5/1 -> Complex Sum1/3
  Complex Sum/1 -> Complex Pole with Mismatch/1
  Complex Pole with Mismatch2/1 -> Complex Sum3/2
  Complex Pole with Mismatch1/1 -> Complex Sum2/2
  Complex Gain7/1 -> Complex Sum3/3
  Complex Gain6/1 -> Complex Sum2/3
  Complex Sum2/1 -> Complex Pole with Mismatch2/1
  Complex Gain3/1 -> Complex Sum3/1
  Complex Gain2/1 -> Complex Sum2/1
  Complex Sum3/1 -> Complex Pole with Mismatch3/1
  Complex Pole with Mismatch3/1 -> Complex Quantizer/1
  Complex Quantizer/1 -> Out1/1, Complex Gain7/1, Complex Gain6/1, Complex Gain5/1, Complex Gain4/1

== system RF/A/D Blocks/5th Order Decimation Filter ==
  Data In : Inport  Port=1
  Downsample : dspbdsp/Downsample  N=N  phase=0  ts=1/fs
  Fifth-Order Integrator : RF/A//D Blocks/Fifth-Order Integrator  fs=fs  N=N
  Data Out : Outport  Port=1  InitialOutput=0
  wires:
  Downsample/1 -> Data Out/1
  Fifth-Order Integrator/1 -> Downsample/1
  Data In/1 -> Fifth-Order Integrator/1

== system RF/A/D Blocks/5th Order  Demodulation and Decimation ==
  D In : Inport  Port=1
  5th Order Decimation Filter : RF/A//D Blocks/5th Order Decimation Filter  N=2*N  fs=fs
  5th Order Decimation Filter1 : RF/A//D Blocks/5th Order Decimation Filter  N=2*N  fs=fs
  Cosine Wave : Sin  Amplitude=1  Frequency=fIF*2*pi  Phase=pi/2  SampleTime=1/fs
  Product : Product  Inputs=2  Multiplication=Element-wise(.*)  SaturateOnIntegerOverflow=on
  Product1 : Product  Inputs=2  Multiplication=Element-wise(.*)  SaturateOnIntegerOverflow=on
  Sine Wave : Sin  Amplitude=-1  Frequency=fIF*2*pi  Phase=0  SampleTime=1/fs
  I Out : Outport  Port=1  InitialOutput=0
  Q Out : Outport  Port=2  InitialOutput=0
  wires:
  Product1/1 -> 5th Order Decimation Filter1/1
  5th Order Decimation Filter1/1 -> Q Out/1
  Product/1 -> 5th Order Decimation Filter/1
  5th Order Decimation Filter/1 -> I Out/1
  Cosine Wave/1 -> Product/1
  Sine Wave/1 -> Product1/2
  D In/1 -> Product/2, Product1/1

== system RF/A/D Blocks/5th Order Complex Demodulation and Decimation ==
  D In : Inport  Port=1
  5th Order Decimation Filter : RF/A//D Blocks/5th Order Decimation Filter  N=N  fs=fs
  5th Order Decimation Filter1 : RF/A//D Blocks/5th Order Decimation Filter  N=N  fs=fs
  Cosine Wave : Sin  Amplitude=1  Frequency=fIF*2*pi  Phase=pi/2  SampleTime=1/fs
  Product{,1..3} (4 alike) : Product  Inputs=2  Multiplication=Element-wise(.*)  SaturateOnIntegerOverflow=on
  Sine Wave : Sin  Amplitude=-1  Frequency=fIF*2*pi  Phase=0  SampleTime=1/fs
  Split : dspcmplx/Split
  Sum : Sum  Inputs=-+  SaturateOnIntegerOverflow=on
  Sum1 : Sum  Inputs=++  SaturateOnIntegerOverflow=on
  I Out : Outport  Port=1  InitialOutput=0
  Q Out : Outport  Port=2  InitialOutput=0
  wires:
  Sum1/1 -> 5th Order Decimation Filter/1
  Sum/1 -> 5th Order Decimation Filter1/1
  5th Order Decimation Filter1/1 -> Q Out/1
  D In/1 -> Split/1
  5th Order Decimation Filter/1 -> I Out/1
  Split/2 -> Product1/1, Product3/1
  Split/1 -> Product/1, Product2/1
  Sine Wave/1 -> Product2/2, Product1/2
  Cosine Wave/1 -> Product3/2, Product/2
  Product/1 -> Sum1/1
  Product1/1 -> Sum1/2
  Product2/1 -> Sum/1
  Product3/1 -> Sum/2

== system RF/A/D Blocks/A/D Converter ==
  In1 : Inport  Port=1
  Constant : Constant  Value=ilevel
  Gain : Gain  Gain=slevel  Multiplication=Element-wise(K.*u)  SaturateOnIntegerOverflow=on
  Quantizer : Quantizer  QuantizationInterval=qlevel  LinearizeAsGain=on
  Rounding Function : Rounding  Operator=round
  Saturation : Saturate  UpperLimit=FSlevel  LowerLimit=0  LinearizeAsGain=on
  Sum : Sum  Inputs=++  SaturateOnIntegerOverflow=on
  Zero-Order Hold : ZeroOrderHold  SampleTime=1/fs
  Out1 : Outport  Port=1  InitialOutput=0
  wires:
  Rounding Function/1 -> Out1/1
  Gain/1 -> Rounding Function/1
  Saturation/1 -> Gain/1
  Quantizer/1 -> Saturation/1
  In1/1 -> Zero-Order Hold/1
  Constant/1 -> Sum/2
  Sum/1 -> Quantizer/1
  Zero-Order Hold/1 -> Sum/1

== system RF/A/D Blocks/Digital Mirror Suppression ==
  I_I : Inport  Port=1
  I_Q : Inport  Port=2
  Q_I : Inport  Port=3
  Q_Q : Inport  Port=4
  Gain : Gain  Gain=g1  Multiplication=Element-wise(K.*u)  SaturateOnIntegerOverflow=on
  Gain1 : Gain  Gain=g2  Multiplication=Element-wise(K.*u)  SaturateOnIntegerOverflow=on
  Sum : Sum  Inputs=++  SaturateOnIntegerOverflow=on
  Sum1 : Sum  Inputs=++  SaturateOnIntegerOverflow=on
  I_Out : Outport  Port=1  InitialOutput=0
  Q_Out : Outport  Port=2  InitialOutput=0
  wires:
  Q_Q/1 -> Sum/2
  Gain/1 -> Sum/1
  I_I/1 -> Gain/1
  Sum/1 -> Q_Out/1
  Gain1/1 -> Sum1/2
  I_Q/1 -> Sum1/1
  Sum1/1 -> I_Out/1
  Q_I/1 -> Gain1/1

== system RF/A/D Blocks/Fifth-Order Integrator ==
  Data In : Inport  Port=1
  Discrete Filter{,1..4} (5 alike) : DiscreteFilter  Numerator=[1 zeros(1,N-1) -1]  Denominator=[1 -1]  SampleTime=1/fs  Realization=auto
  Gain{,1..4} (5 alike) : Gain  Gain=1/N  Multiplication=Element-wise(K.*u)  SaturateOnIntegerOverflow=on
  Data Out : Outport  Port=1  InitialOutput=0
  wires:
  Gain4/1 -> Data Out/1
  Gain/1 -> Discrete Filter1/1
  Gain3/1 -> Discrete Filter4/1
  Discrete Filter4/1 -> Gain4/1
  Discrete Filter3/1 -> Gain3/1
  Gain2/1 -> Discrete Filter3/1
  Discrete Filter2/1 -> Gain2/1
  Gain1/1 -> Discrete Filter2/1
  Discrete Filter1/1 -> Gain1/1
  Discrete Filter/1 -> Gain/1
  Data In/1 -> Discrete Filter/1
